simulink model "HW3"  (R2016b)
settings: Solver=FixedStepAuto  StartTime=0.0  StopTime=1  FixedStep=0.01  RelTol=1e-3
libraries: fuzblock x1
settings Model: Creator=Minh  LastModifiedBy=Minh
settings DataIOCC: LimitDataPoints=on  SaveOutput=off  SaveTime=off
settings OptimizationCC: BlockReduction=off  BooleanDataType=off  LifeSpan=inf
settings DebuggingCC: SaveWithParameterizedLinksMsg=none  UnderspecifiedInitializationDetection=Classic  MergeDetectMultiDrivingBlocksExec=none  SignalResolutionControl=TryResolveAllWithWarning  AllowSymbolicDim=off  SFUnexpectedBacktrackingDiag=warning  SFNoUnconditionalDefaultTransitionDiag=warning  SFExecutionAtInitializationDiag=none
settings HardwareCC: TargetUnknown=on
settings GRTTargetCC: TargetLangStandard=C89/C90 (ANSI)  GeneratePreprocessorConditionals=Disable all
settings ConfigComp: CovMetricSettings=dw  CovHtmlReporting=on  CovSaveCumulativeToWorkspaceVar=on  CovSaveSingleToWorkspaceVar=on  CovExternalEMLEnable=off

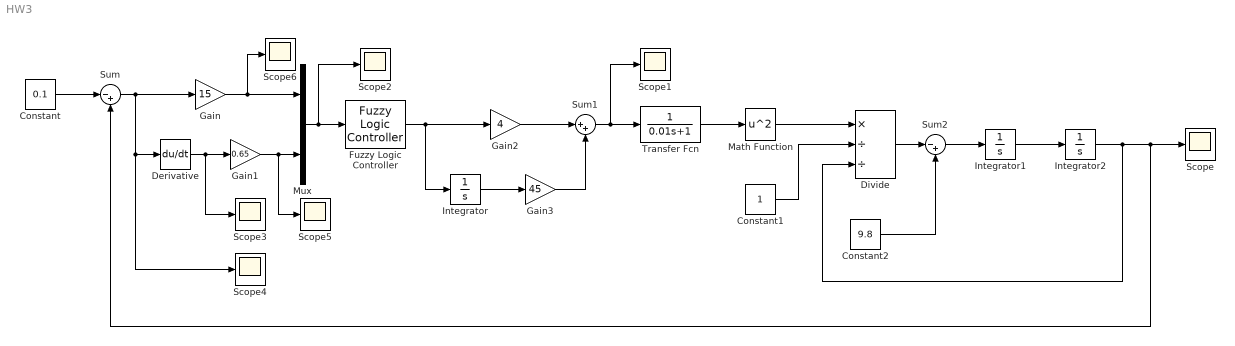
== system HW3 ==
  Constant : Constant  Value=0.1  SampleTime=0.01
  Constant1 : Constant  SampleTime=0.01
  Constant2 : Constant  Value=9.8  SampleTime=0.01
  Derivative : Derivative
  Divide : Product  Inputs=*//
  Fuzzy Logic Controller : fuzblock/Fuzzy Logic  Controller  fis='flc.fis'
  Gain : Gain  Gain=15
  Gain1 : Gain  Gain=0.65
  Gain2 : Gain  Gain=4
  Gain3 : Gain  Gain=45
  Integrator : Integrator
  Integrator1 : Integrator
  Integrator2 : Integrator  InitialCondition=0.1
  Math Function : Math  Operator=square  SaturateOnIntegerOverflow=on
  Mux : Mux  Inputs=2
  Scope{,1..6} (7 alike) : Scope
  Sum : Sum  Inputs=|-+
  Sum1 : Sum  Inputs=|++
  Sum2 : Sum  Inputs=|-+
  Transfer Fcn : TransferFcn  Denominator=[0.01 1]
  wires:
  Constant/1 -> Sum/1
  Sum/1 -> Scope4/1, Derivative/1, Gain/1
  Derivative/1 -> Scope3/1, Gain1/1
  Gain/1 -> Scope6/1, Mux/1
  Gain1/1 -> Scope5/1, Mux/2
  Mux/1 -> Scope2/1, Fuzzy Logic Controller/1
  Fuzzy Logic Controller/1 -> Integrator/1, Gain2/1
  Integrator/1 -> Gain3/1
  Gain2/1 -> Sum1/1
  Gain3/1 -> Sum1/2
  Sum1/1 -> Scope1/1, Transfer Fcn/1
  Transfer Fcn/1 -> Math Function/1
  Math Function/1 -> Divide/1
  Constant1/1 -> Divide/2
  Divide/1 -> Sum2/1
  Sum2/1 -> Integrator1/1
  Integrator1/1 -> Integrator2/1
  Constant2/1 -> Sum2/2
  Integrator2/1 -> Scope/1, Sum/2, Divide/3
